simulink model "combinedTxRx_ADIDMA"  (R2017b)
settings: Solver=FixedStepDiscrete  StartTime=0.0  StopTime=10.0  RelTol=1e-3
InitFcn:
  | modelSettings
undefined symbols (not defined in the file or in its folder): RadioSampleRate
libraries: RxTxFixedPointLibrary_noscopes x2, dspsigops x2, commsource2 x1, simulink x1, commfilt2 x1
settings Model: Creator=tcollins  LastModifiedBy=tcollins
settings OptimizationCC: BlockReduction=off  ConditionallyExecuteInputs=off  DefaultParameterBehavior=Inlined
settings DebuggingCC: AlgebraicLoopMsg=error  SingleTaskRateTransMsg=error
settings HardwareCC: ProdBitPerPointer=32  ProdBitPerSizeT=32  ProdBitPerPtrDiffT=32  ProdLargestAtomicFloat=None  ProdIntDivRoundTo=Undefined  ProdEndianess=Unspecified  ProdWordSize=32  ProdHWDeviceType=ASIC/FPGA->ASIC/FPGA  ProdEqTarget=off
settings CodeAppCC: StateflowObjectComments=on

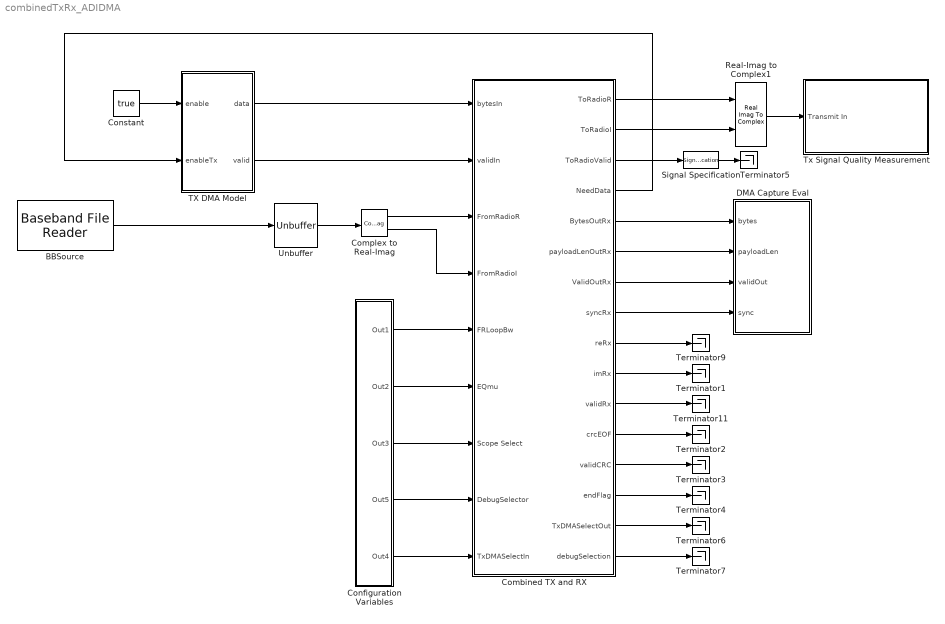
== system combinedTxRx_ADIDMA ==
  BBSource : commsource2/Baseband File Reader  Filename=PlutoCaptureQPSK.bb  InheritSampleTimeFromFile=off  SampleTime=100000/(RadioSampleRate)  SamplesPerFrame=100000  CyclicRepetition=off  FileEndOutputPort=off  SimulateUsing=Interpreted execution
      settings: SourceProductName=Communications System Toolbox  SourceProductBaseCode=CM
  Combined TX and RX : Subsystem  TreatAsAtomicUnit=on
  Complex to Real-Imag : ComplexToRealImag
  Configuration Variables : Subsystem
  Constant : Constant  Value=true  SampleTime=-1
  DMA Capture Eval : MATLAB Function  TreatAsAtomicUnit=on
  Real-Imag to Complex1 : RealImagToComplex
  Signal Specification : SignalSpecification  SampleTime=1/RadioSampleRate
  TX DMA Model : Subsystem
  Terminator{1..7,9,11} (9 alike) : Terminator
  Tx Signal Quality Measurement : Subsystem
  Unbuffer : Unbuffer
  wires:
  BBSource/1 -> Unbuffer/1
  Unbuffer/1 -> Complex to Real-Imag/1
  Complex to Real-Imag/1 -> Combined TX and RX/3(FromRadioR)
  Complex to Real-Imag/2 -> Combined TX and RX/4(FromRadioI)
  Combined TX and RX/1(ToRadioR) -> Real-Imag to Complex1/1
  Combined TX and RX/2(ToRadioI) -> Real-Imag to Complex1/2
  Combined TX and RX/3(ToRadioValid) -> Signal Specification/1
  Combined TX and RX/5(BytesOutRx) -> DMA Capture Eval/1(bytes)
  Combined TX and RX/6(payloadLenOutRx) -> DMA Capture Eval/2(payloadLen)
  Combined TX and RX/8(syncRx) -> DMA Capture Eval/4(sync)
  Combined TX and RX/11(validRx) -> Terminator11/1
  Real-Imag to Complex1/1 -> Tx Signal Quality Measurement/1(Transmit In)
  Configuration Variables/3(Out3) -> Combined TX and RX/7(Scope Select)
  Configuration Variables/1(Out1) -> Combined TX and RX/5(FRLoopBw)
  Configuration Variables/2(Out2) -> Combined TX and RX/6(EQmu)
  Combined TX and RX/7(ValidOutRx) -> DMA Capture Eval/3(validOut)
  Constant/1 -> TX DMA Model/1(enable)
  Combined TX and RX/4(NeedData) -> TX DMA Model/2(enableTx)
  TX DMA Model/1(data) -> Combined TX and RX/1(bytesIn)
  TX DMA Model/2(valid) -> Combined TX and RX/2(validIn)
  Combined TX and RX/9(reRx) -> Terminator9/1
  Combined TX and RX/10(imRx) -> Terminator1/1
  Combined TX and RX/12(crcEOF) -> Terminator2/1
  Combined TX and RX/13(validCRC) -> Terminator3/1
  Combined TX and RX/14(endFlag) -> Terminator4/1
  Combined TX and RX/15(TxDMASelectOut) -> Terminator6/1
  Combined TX and RX/16(debugSelection) -> Terminator7/1
  Configuration Variables/4(Out5) -> Combined TX and RX/8(DebugSelector)
  Configuration Variables/5(Out4) -> Combined TX and RX/9(TxDMASelectIn)
  Signal Specification/1 -> Terminator5/1

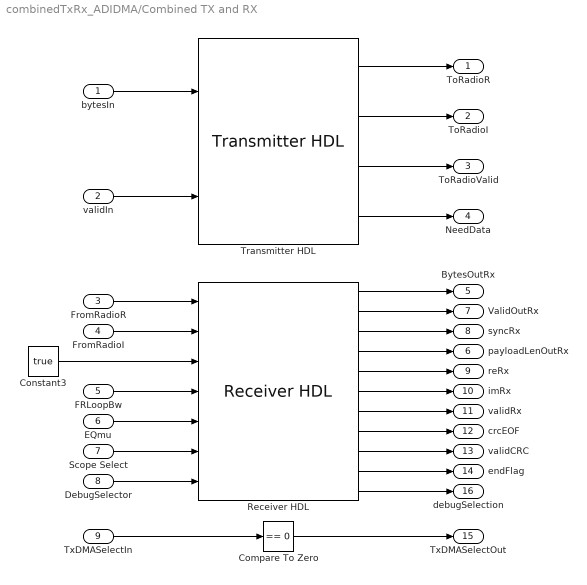
== system combinedTxRx_ADIDMA/Combined TX and RX ==
  bytesIn : Inport
  validIn : Inport  Port=2
  FromRadioR : Inport  Port=3
  FromRadioI : Inport  Port=4
  FRLoopBw : Inport  Port=5
  EQmu : Inport  Port=6
  Scope Select : Inport  Port=7
  DebugSelector : Inport  Port=8
  TxDMASelectIn : Inport  Port=9
  Compare To Zero : simulink/Logic and Bit Operations/Compare To Zero  relop===  OutDataTypeStr=boolean
  Constant3 : Constant  Value=true  SampleTime=1/RadioSampleRate
  Receiver HDL : RxTxFixedPointLibrary_noscopes/Receiver HDL  SystemSampleTime=-1
  Transmitter HDL : RxTxFixedPointLibrary_noscopes/Transmitter HDL  SystemSampleTime=-1
  ToRadioR : Outport
  ToRadioI : Outport  Port=2
  ToRadioValid : Outport  Port=3
  NeedData : Outport  Port=4
  BytesOutRx : Outport  Port=5
  payloadLenOutRx : Outport  Port=6
  ValidOutRx : Outport  Port=7
  syncRx : Outport  Port=8
  reRx : Outport  Port=9
  imRx : Outport  Port=10
  validRx : Outport  Port=11
  crcEOF : Outport  Port=12
  validCRC : Outport  Port=13
  endFlag : Outport  Port=14
  TxDMASelectOut : Outport  Port=15
  debugSelection : Outport  Port=16
  wires:
  Receiver HDL/2 -> ValidOutRx/1
  Receiver HDL/3 -> syncRx/1
  Receiver HDL/7 -> validRx/1
  Receiver HDL/5 -> reRx/1
  Receiver HDL/1 -> BytesOutRx/1
  validIn/1 -> Transmitter HDL/2
  Transmitter HDL/2 -> ToRadioI/1
  Transmitter HDL/3 -> ToRadioValid/1
  Transmitter HDL/1 -> ToRadioR/1
  bytesIn/1 -> Transmitter HDL/1
  Transmitter HDL/4 -> NeedData/1
  FromRadioR/1 -> Receiver HDL/1
  FromRadioI/1 -> Receiver HDL/2
  Constant3/1 -> Receiver HDL/3
  FRLoopBw/1 -> Receiver HDL/4
  EQmu/1 -> Receiver HDL/5
  Scope Select/1 -> Receiver HDL/6
  Receiver HDL/4 -> payloadLenOutRx/1
  Receiver HDL/6 -> imRx/1
  Receiver HDL/8 -> crcEOF/1
  Receiver HDL/9 -> validCRC/1
  Receiver HDL/10 -> endFlag/1
  TxDMASelectIn/1 -> Compare To Zero/1
  Compare To Zero/1 -> TxDMASelectOut/1
  DebugSelector/1 -> Receiver HDL/7
  Receiver HDL/11 -> debugSelection/1

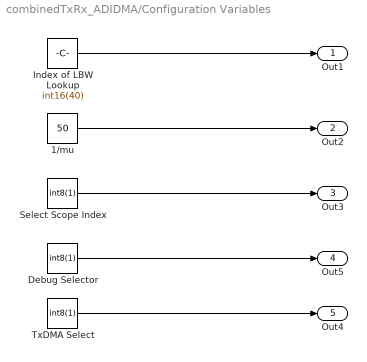
== system combinedTxRx_ADIDMA/Configuration Variables ==
  1/mu : Constant  Value=50  OutDataTypeStr=int16  SampleTime=-1
  Debug Selector : Constant  Value=int8(1)  SampleTime=1/RadioSampleRate
  Index of LBW Lookup : Constant  Value=int16(40)  SampleTime=1/RadioSampleRate
  Select Scope Index : Constant  Value=int8(1)  SampleTime=1/RadioSampleRate
  TxDMA Select : Constant  Value=int8(1)  SampleTime=1/RadioSampleRate
  Out1 : Outport
  Out2 : Outport  Port=2
  Out3 : Outport  Port=3
  Out5 : Outport  Port=4
  Out4 : Outport  Port=5
  wires:
  1/mu/1 -> Out2/1
  Index of LBW Lookup/1 -> Out1/1
  Select Scope Index/1 -> Out3/1
  TxDMA Select/1 -> Out4/1
  Debug Selector/1 -> Out5/1

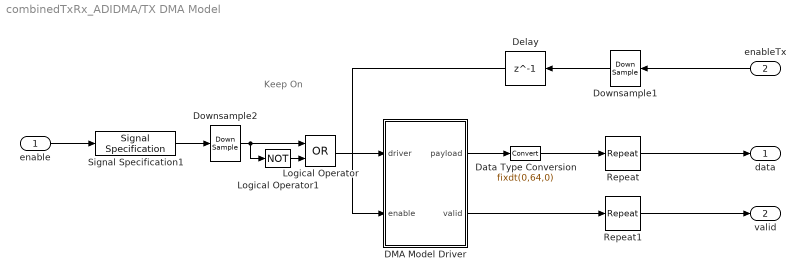
== system combinedTxRx_ADIDMA/TX DMA Model ==
  note: Keep On
  enable : Inport
  enableTx : Inport  Port=2
  DMA Model Driver : MATLAB Function  TreatAsAtomicUnit=on
  Data Type Conversion : DataTypeConversion  OutDataTypeStr=fixdt(0,64,0)
  Delay : Delay  DelayLength=1
  Downsample1 : DownSample  N=4  RateOptions=Allow multirate processing
  Downsample2 : DownSample  N=4  RateOptions=Allow multirate processing
  Logical Operator : Logic  Operator=OR  AllPortsSameDT=off  OutDataTypeStr=boolean
  Logical Operator1 : Logic  Operator=NOT  AllPortsSameDT=off  OutDataTypeStr=boolean
  Repeat : dspsigops/Repeat  N=4  InputProcessing=Columns as channels (frame based)  RateOptions=Allow multirate processing  ic=0  mode=Unused parameter value
      settings: SourceProductName=DSP System Toolbox
  Repeat1 : dspsigops/Repeat  N=4  InputProcessing=Columns as channels (frame based)  RateOptions=Allow multirate processing  ic=0  mode=Unused parameter value
      settings: SourceProductName=DSP System Toolbox
  Signal Specification1 : SignalSpecification  OutDataTypeStr=boolean  SampleTime=1e-6
  data : Outport
  valid : Outport  Port=2
  wires:
  Downsample2/1 -> Logical Operator/1, Logical Operator1/1
  Logical Operator/1 -> DMA Model Driver/1(driver)
  Repeat1/1 -> valid/1
  DMA Model Driver/2(valid) -> Repeat1/1
  enableTx/1 -> Downsample1/1
  Data Type Conversion/1 -> Repeat/1
  Downsample1/1 -> Delay/1
  Signal Specification1/1 -> Downsample2/1
  Delay/1 -> DMA Model Driver/2(enable)
  Logical Operator1/1 -> Logical Operator/2
  DMA Model Driver/1(payload) -> Data Type Conversion/1
  enable/1 -> Signal Specification1/1
  Repeat/1 -> data/1

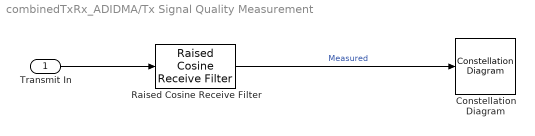
== system combinedTxRx_ADIDMA/Tx Signal Quality Measurement ==
  Transmit In : Inport
  Constellation Diagram : ConstellationDiagram
  Raised Cosine Receive Filter : commfilt2/Raised Cosine Receive Filter  filtType=Square root  R=0.5  filtSpan=8  N=4  downFactor=4  downOffset=0  filterGain=1  RateOptions=Allow multirate processing  framing=Mute  checkCoeff=off  variableName=rcRxFilt  currentFiltSpan=8  D=(8)/2  inputOffset=0  sampMode=Mute  saveAsFlag=0  rateMode=Downsampling  checkGain=Normalized  launchFVT=on  roundingMode=Floor  overflowMode=off  coeffDataTypeStr=Inherit: Same word length as input  coeffMin=[]  coeffMax=[]  coeffLastDataTypeStr=Inherit: Same word length as input  accumDataTypeStr=Inherit: Same as product output  accumLastDataTypeStr=Inherit: Same as product output  outputDataTypeStr=Inherit: Same as accumulator  outputMin=[]  outputMax=[]  outputLastDataTypeStr=Inherit: Same as accumulator
  wires:
  Transmit In/1 -> Raised Cosine Receive Filter/1
  Raised Cosine Receive Filter/1 -> Constellation Diagram/1  "Measured"

== matlab function combinedTxRx_ADIDMA/DMA Capture Eval ==
  data: bytes input; payloadLen input; validOut input; sync input
function fcn(bytes, payloadLen, validOut, sync)

persistent frameBuffer byteCounter fullPayloadBits

bitsInPack = 64;

if isempty(frameBuffer)
    maxFrameBits = (2^16)*8;
    frameBuffer = false(maxFrameBits,1);
    byteCounter = 0;
    fullPayloadBits = uint16(0);
end

if validOut
    if sync
        byteCounter = bitsInPack;
        frameBuffer(1:byteCounter) = bitget(bytes,1:bitsInPack);
        fullPayloadBits = uint16(payloadLen*8);
        
    elseif byteCounter<fullPayloadBits
        frameBuffer(byteCounter+1:byteCounter+bitsInPack) = bitget(bytes,1:bitsInPack);
        byteCounter = byteCounter + bitsInPack;
    else
        if bytes>0
            disp('CRC Error (Outside)');
        else
            disp('Frame passed CRC (Outside)');
        end
    end
end

== matlab function combinedTxRx_ADIDMA/TX DMA Model/DMA Model Driver ==
  data: driver input; payload output; valid output boolean; enable input
function [payload,valid] = fcn(driver, enable)
%#codegen

persistent indx mode

pSize = fi(200,0,64,0); % Size in bytes (Must be multiple of 32 bits) cannot exceed uint16 max
mask = uint16(sum(2.^(0:15)));

if isempty(indx)
    indx = pSize;
    mode = int8(0);
end

% % Randomly dont transmit new data
% if enable && mode == 0
%    enable = randn>1; 
% end

if enable && driver
    valid = true;
    switch mode
        case int8(0) % Fresh packet start
%             disp('New Packet Start');
            payload = fi(pSize,0,64,0);%Upper bits
            mode = int8(1);
            indx = fi(0,0,64,0);
        otherwise%case 2
            indx = fi(indx + fi(8,0,64,0),0,64,0);
            %payload = uint32(sum(2.^[0 2 4 6 8 10 12 14 ]));
            if indx == fi(8,0,64,0)
                payload = fi(0,0,64,0);
            elseif indx == pSize
                payload = fi(uint64(18446744073709551615),0,64,0); % All ones
            else
                payload = fi(uint64(12297829382473034410),0,64,0);%sum(2.^[0:2:14])); % Alternating ones and zeros
            end
            
            if indx == pSize % reached end of frame
                mode = int8(0);
            end
    end
else
    valid = false;
    payload = fi(0,0,64,0);
end
